simulink model "c960x4096_x14_7_r2013b_frb"  (R2013b)
settings: Solver=ode45  StartTime=0.0  StopTime=40960  RelTol=1e-3
undefined symbols (not defined in the file): sfp
libraries: xbsIndex_r4 x14620, casper_library_misc x61, dspsigops x32, casper_library_multipliers x24, simulink x18, xps_library x18
(part 17 of 79)

== system c960x4096_x14_7_r2013b_frb/ds_to_tgbe/mb1/mb_5 ==
  DIN_0 : Inport
  DIN_1 : Inport  Port=2
  DIN_2 : Inport  Port=3
  DIN_3 : Inport  Port=4
  W_ADDR : Inport  Port=5
  R_ADDR : Inport  Port=6
  WE : Inport  Port=7
  MUX_SEL : Inport  Port=8
  Concat{,1..3} (4 alike) : xbsIndex_r4/Concat  num_inputs=2  dbl_ovrd=off  block_type=concat
  Mux1 : xbsIndex_r4/Mux  inputs=4  en=off  latency=0  precision=Full  arith_type=Unsigned  n_bits=16  bin_pt=14  quantization=Truncate  overflow=Wrap  dbl_ovrd=off  block_type=mux
  Mux2 : xbsIndex_r4/Mux  inputs=2  en=off  latency=0  precision=Full  arith_type=Unsigned  n_bits=16  bin_pt=14  quantization=Truncate  overflow=Wrap  dbl_ovrd=off  block_type=mux
  Slice_Data_0 : Subsystem
  Slice_Data_1 : Subsystem
  Slice_Data_2 : Subsystem
  Slice_Data_3 : Subsystem
  b0h : Subsystem  Tag=xps:bram  AncestorBlock=xps_library/Shared BRAM  mask{arith_type=Unsigned, addr_width=10, data_width=32, reg_prim_output=off, reg_core_output=off, optimization=Minimum_Area, data_bin_pt=0, init_vals=[0:0], sample_rate=1}
      mask prompts: arith_type "Output Data Type"; addr_width "Address width"; data_width "Data Width"; reg_prim_output "Register Primitive Output"; reg_core_output "Register Core Output"; data_bin_pt "Data Binary Point"; init_vals "Initial values (simulation only)"; sample_rate "Sample rate"
      mask init:
      | shared_bram_mask;
      mask TypeOptions arith_type: Unsigned | Signed  (2's comp)
      mask TypeOptions data_width: 8 | 16 | 32 | 64 | 128
      mask TypeOptions optimization: Minimum_Area | Low_Power
  b0l : Subsystem  Tag=xps:bram  AncestorBlock=xps_library/Shared BRAM  mask{arith_type=Unsigned, addr_width=10, data_width=32, reg_prim_output=off, reg_core_output=off, optimization=Minimum_Area, data_bin_pt=0, init_vals=[0:0], sample_rate=1}
      mask prompts: arith_type "Output Data Type"; addr_width "Address width"; data_width "Data Width"; reg_prim_output "Register Primitive Output"; reg_core_output "Register Core Output"; data_bin_pt "Data Binary Point"; init_vals "Initial values (simulation only)"; sample_rate "Sample rate"
      mask init:
      | shared_bram_mask;
      mask TypeOptions arith_type: Unsigned | Signed  (2's comp)
      mask TypeOptions data_width: 8 | 16 | 32 | 64 | 128
      mask TypeOptions optimization: Minimum_Area | Low_Power
  b1h : Subsystem  Tag=xps:bram  AncestorBlock=xps_library/Shared BRAM  mask{arith_type=Unsigned, addr_width=10, data_width=32, reg_prim_output=off, reg_core_output=off, optimization=Minimum_Area, data_bin_pt=0, init_vals=[0:0], sample_rate=1}
      mask prompts: arith_type "Output Data Type"; addr_width "Address width"; data_width "Data Width"; reg_prim_output "Register Primitive Output"; reg_core_output "Register Core Output"; data_bin_pt "Data Binary Point"; init_vals "Initial values (simulation only)"; sample_rate "Sample rate"
      mask init:
      | shared_bram_mask;
      mask TypeOptions arith_type: Unsigned | Signed  (2's comp)
      mask TypeOptions data_width: 8 | 16 | 32 | 64 | 128
      mask TypeOptions optimization: Minimum_Area | Low_Power
  b1l : Subsystem  Tag=xps:bram  AncestorBlock=xps_library/Shared BRAM  mask{arith_type=Unsigned, addr_width=10, data_width=32, reg_prim_output=off, reg_core_output=off, optimization=Minimum_Area, data_bin_pt=0, init_vals=[0:0], sample_rate=1}
      mask prompts: arith_type "Output Data Type"; addr_width "Address width"; data_width "Data Width"; reg_prim_output "Register Primitive Output"; reg_core_output "Register Core Output"; data_bin_pt "Data Binary Point"; init_vals "Initial values (simulation only)"; sample_rate "Sample rate"
      mask init:
      | shared_bram_mask;
      mask TypeOptions arith_type: Unsigned | Signed  (2's comp)
      mask TypeOptions data_width: 8 | 16 | 32 | 64 | 128
      mask TypeOptions optimization: Minimum_Area | Low_Power
  b2h : Subsystem  Tag=xps:bram  AncestorBlock=xps_library/Shared BRAM  mask{arith_type=Unsigned, addr_width=10, data_width=32, reg_prim_output=off, reg_core_output=off, optimization=Minimum_Area, data_bin_pt=0, init_vals=[0:0], sample_rate=1}
      mask prompts: arith_type "Output Data Type"; addr_width "Address width"; data_width "Data Width"; reg_prim_output "Register Primitive Output"; reg_core_output "Register Core Output"; data_bin_pt "Data Binary Point"; init_vals "Initial values (simulation only)"; sample_rate "Sample rate"
      mask init:
      | shared_bram_mask;
      mask TypeOptions arith_type: Unsigned | Signed  (2's comp)
      mask TypeOptions data_width: 8 | 16 | 32 | 64 | 128
      mask TypeOptions optimization: Minimum_Area | Low_Power
  b2l : Subsystem  Tag=xps:bram  AncestorBlock=xps_library/Shared BRAM  mask{arith_type=Unsigned, addr_width=10, data_width=32, reg_prim_output=off, reg_core_output=off, optimization=Minimum_Area, data_bin_pt=0, init_vals=[0:0], sample_rate=1}
      mask prompts: arith_type "Output Data Type"; addr_width "Address width"; data_width "Data Width"; reg_prim_output "Register Primitive Output"; reg_core_output "Register Core Output"; data_bin_pt "Data Binary Point"; init_vals "Initial values (simulation only)"; sample_rate "Sample rate"
      mask init:
      | shared_bram_mask;
      mask TypeOptions arith_type: Unsigned | Signed  (2's comp)
      mask TypeOptions data_width: 8 | 16 | 32 | 64 | 128
      mask TypeOptions optimization: Minimum_Area | Low_Power
  b3h : Subsystem  Tag=xps:bram  AncestorBlock=xps_library/Shared BRAM  mask{arith_type=Unsigned, addr_width=10, data_width=32, reg_prim_output=off, reg_core_output=off, optimization=Minimum_Area, data_bin_pt=0, init_vals=[0:0], sample_rate=1}
      mask prompts: arith_type "Output Data Type"; addr_width "Address width"; data_width "Data Width"; reg_prim_output "Register Primitive Output"; reg_core_output "Register Core Output"; data_bin_pt "Data Binary Point"; init_vals "Initial values (simulation only)"; sample_rate "Sample rate"
      mask init:
      | shared_bram_mask;
      mask TypeOptions arith_type: Unsigned | Signed  (2's comp)
      mask TypeOptions data_width: 8 | 16 | 32 | 64 | 128
      mask TypeOptions optimization: Minimum_Area | Low_Power
  b3l : Subsystem  Tag=xps:bram  AncestorBlock=xps_library/Shared BRAM  mask{arith_type=Unsigned, addr_width=10, data_width=32, reg_prim_output=off, reg_core_output=off, optimization=Minimum_Area, data_bin_pt=0, init_vals=[0:0], sample_rate=1}
      mask prompts: arith_type "Output Data Type"; addr_width "Address width"; data_width "Data Width"; reg_prim_output "Register Primitive Output"; reg_core_output "Register Core Output"; data_bin_pt "Data Binary Point"; init_vals "Initial values (simulation only)"; sample_rate "Sample rate"
      mask init:
      | shared_bram_mask;
      mask TypeOptions arith_type: Unsigned | Signed  (2's comp)
      mask TypeOptions data_width: 8 | 16 | 32 | 64 | 128
      mask TypeOptions optimization: Minimum_Area | Low_Power
  DOUT : Outport
  wires:
  b0h/1(data_out) -> Concat/1
  [R_ADDR] -> Mux2/2
  [W_ADDR] -> Mux2/3
  [WE] -> Mux2/1
  Mux2/1 -> [ADDR]
  R_ADDR/1 -> [R_ADDR]
  Mux1/1 -> DOUT/1
  Concat3/1 -> [MB_3]
  Concat2/1 -> [MB_2]
  Concat1/1 -> [MB_1]
  Concat/1 -> [MB_0]
  [MB_3] -> Mux1/5
  [MB_2] -> Mux1/4
  [MB_1] -> Mux1/3
  [MB_0] -> Mux1/2
  [MUX_SEL] -> Mux1/1
  [ADDR] -> b3l/1(addr), b3h/1(addr), b2l/1(addr), b2h/1(addr), b1l/1(addr), b1h/1(addr), b0l/1(addr), b0h/1(addr)
  [DIN_3] -> Slice_Data_3/1(DIN)
  [DIN_2] -> Slice_Data_2/1(DIN)
  [DIN_1] -> Slice_Data_1/1(DIN)
  [DIN_0] -> Slice_Data_0/1(DIN)
  Slice_Data_3/2(DOUT_LO) -> b3l/2(data_in)
  Slice_Data_3/1(DOUT_HI) -> b3h/2(data_in)
  Slice_Data_2/2(DOUT_LO) -> b2l/2(data_in)
  Slice_Data_2/1(DOUT_HI) -> b2h/2(data_in)
  Slice_Data_1/2(DOUT_LO) -> b1l/2(data_in)
  Slice_Data_1/1(DOUT_HI) -> b1h/2(data_in)
  Slice_Data_0/2(DOUT_LO) -> b0l/2(data_in)
  Slice_Data_0/1(DOUT_HI) -> b0h/2(data_in)
  [WE] -> b3l/3(we), b3h/3(we), b2l/3(we), b2h/3(we), b1l/3(we), b1h/3(we), b0l/3(we), b0h/3(we)
  b3l/1(data_out) -> Concat3/2
  b3h/1(data_out) -> Concat3/1
  b2l/1(data_out) -> Concat2/2
  b2h/1(data_out) -> Concat2/1
  b1l/1(data_out) -> Concat1/2
  b1h/1(data_out) -> Concat1/1
  b0l/1(data_out) -> Concat/2
  MUX_SEL/1 -> [MUX_SEL]
  WE/1 -> [WE]
  W_ADDR/1 -> [W_ADDR]
  DIN_3/1 -> [DIN_3]
  DIN_2/1 -> [DIN_2]
  DIN_1/1 -> [DIN_1]
  DIN_0/1 -> [DIN_0]

== system c960x4096_x14_7_r2013b_frb/ds_to_tgbe/mb1/mb_6 ==
  DIN_0 : Inport
  DIN_1 : Inport  Port=2
  DIN_2 : Inport  Port=3
  DIN_3 : Inport  Port=4
  W_ADDR : Inport  Port=5
  R_ADDR : Inport  Port=6
  WE : Inport  Port=7
  MUX_SEL : Inport  Port=8
  Concat{,1..3} (4 alike) : xbsIndex_r4/Concat  num_inputs=2  dbl_ovrd=off  block_type=concat
  Mux1 : xbsIndex_r4/Mux  inputs=4  en=off  latency=0  precision=Full  arith_type=Unsigned  n_bits=16  bin_pt=14  quantization=Truncate  overflow=Wrap  dbl_ovrd=off  block_type=mux
  Mux2 : xbsIndex_r4/Mux  inputs=2  en=off  latency=0  precision=Full  arith_type=Unsigned  n_bits=16  bin_pt=14  quantization=Truncate  overflow=Wrap  dbl_ovrd=off  block_type=mux
  Slice_Data_0 : Subsystem
  Slice_Data_1 : Subsystem
  Slice_Data_2 : Subsystem
  Slice_Data_3 : Subsystem
  b0h : Subsystem  Tag=xps:bram  AncestorBlock=xps_library/Shared BRAM  mask{arith_type=Unsigned, addr_width=10, data_width=32, reg_prim_output=off, reg_core_output=off, optimization=Minimum_Area, data_bin_pt=0, init_vals=[0:0], sample_rate=1}
      mask prompts: arith_type "Output Data Type"; addr_width "Address width"; data_width "Data Width"; reg_prim_output "Register Primitive Output"; reg_core_output "Register Core Output"; data_bin_pt "Data Binary Point"; init_vals "Initial values (simulation only)"; sample_rate "Sample rate"
      mask init:
      | shared_bram_mask;
      mask TypeOptions arith_type: Unsigned | Signed  (2's comp)
      mask TypeOptions data_width: 8 | 16 | 32 | 64 | 128
      mask TypeOptions optimization: Minimum_Area | Low_Power
  b0l : Subsystem  Tag=xps:bram  AncestorBlock=xps_library/Shared BRAM  mask{arith_type=Unsigned, addr_width=10, data_width=32, reg_prim_output=off, reg_core_output=off, optimization=Minimum_Area, data_bin_pt=0, init_vals=[0:0], sample_rate=1}
      mask prompts: arith_type "Output Data Type"; addr_width "Address width"; data_width "Data Width"; reg_prim_output "Register Primitive Output"; reg_core_output "Register Core Output"; data_bin_pt "Data Binary Point"; init_vals "Initial values (simulation only)"; sample_rate "Sample rate"
      mask init:
      | shared_bram_mask;
      mask TypeOptions arith_type: Unsigned | Signed  (2's comp)
      mask TypeOptions data_width: 8 | 16 | 32 | 64 | 128
      mask TypeOptions optimization: Minimum_Area | Low_Power
  b1h : Subsystem  Tag=xps:bram  AncestorBlock=xps_library/Shared BRAM  mask{arith_type=Unsigned, addr_width=10, data_width=32, reg_prim_output=off, reg_core_output=off, optimization=Minimum_Area, data_bin_pt=0, init_vals=[0:0], sample_rate=1}
      mask prompts: arith_type "Output Data Type"; addr_width "Address width"; data_width "Data Width"; reg_prim_output "Register Primitive Output"; reg_core_output "Register Core Output"; data_bin_pt "Data Binary Point"; init_vals "Initial values (simulation only)"; sample_rate "Sample rate"
      mask init:
      | shared_bram_mask;
      mask TypeOptions arith_type: Unsigned | Signed  (2's comp)
      mask TypeOptions data_width: 8 | 16 | 32 | 64 | 128
      mask TypeOptions optimization: Minimum_Area | Low_Power
  b1l : Subsystem  Tag=xps:bram  AncestorBlock=xps_library/Shared BRAM  mask{arith_type=Unsigned, addr_width=10, data_width=32, reg_prim_output=off, reg_core_output=off, optimization=Minimum_Area, data_bin_pt=0, init_vals=[0:0], sample_rate=1}
      mask prompts: arith_type "Output Data Type"; addr_width "Address width"; data_width "Data Width"; reg_prim_output "Register Primitive Output"; reg_core_output "Register Core Output"; data_bin_pt "Data Binary Point"; init_vals "Initial values (simulation only)"; sample_rate "Sample rate"
      mask init:
      | shared_bram_mask;
      mask TypeOptions arith_type: Unsigned | Signed  (2's comp)
      mask TypeOptions data_width: 8 | 16 | 32 | 64 | 128
      mask TypeOptions optimization: Minimum_Area | Low_Power
  b2h : Subsystem  Tag=xps:bram  AncestorBlock=xps_library/Shared BRAM  mask{arith_type=Unsigned, addr_width=10, data_width=32, reg_prim_output=off, reg_core_output=off, optimization=Minimum_Area, data_bin_pt=0, init_vals=[0:0], sample_rate=1}
      mask prompts: arith_type "Output Data Type"; addr_width "Address width"; data_width "Data Width"; reg_prim_output "Register Primitive Output"; reg_core_output "Register Core Output"; data_bin_pt "Data Binary Point"; init_vals "Initial values (simulation only)"; sample_rate "Sample rate"
      mask init:
      | shared_bram_mask;
      mask TypeOptions arith_type: Unsigned | Signed  (2's comp)
      mask TypeOptions data_width: 8 | 16 | 32 | 64 | 128
      mask TypeOptions optimization: Minimum_Area | Low_Power
  b2l : Subsystem  Tag=xps:bram  AncestorBlock=xps_library/Shared BRAM  mask{arith_type=Unsigned, addr_width=10, data_width=32, reg_prim_output=off, reg_core_output=off, optimization=Minimum_Area, data_bin_pt=0, init_vals=[0:0], sample_rate=1}
      mask prompts: arith_type "Output Data Type"; addr_width "Address width"; data_width "Data Width"; reg_prim_output "Register Primitive Output"; reg_core_output "Register Core Output"; data_bin_pt "Data Binary Point"; init_vals "Initial values (simulation only)"; sample_rate "Sample rate"
      mask init:
      | shared_bram_mask;
      mask TypeOptions arith_type: Unsigned | Signed  (2's comp)
      mask TypeOptions data_width: 8 | 16 | 32 | 64 | 128
      mask TypeOptions optimization: Minimum_Area | Low_Power
  b3h : Subsystem  Tag=xps:bram  AncestorBlock=xps_library/Shared BRAM  mask{arith_type=Unsigned, addr_width=10, data_width=32, reg_prim_output=off, reg_core_output=off, optimization=Minimum_Area, data_bin_pt=0, init_vals=[0:0], sample_rate=1}
      mask prompts: arith_type "Output Data Type"; addr_width "Address width"; data_width "Data Width"; reg_prim_output "Register Primitive Output"; reg_core_output "Register Core Output"; data_bin_pt "Data Binary Point"; init_vals "Initial values (simulation only)"; sample_rate "Sample rate"
      mask init:
      | shared_bram_mask;
      mask TypeOptions arith_type: Unsigned | Signed  (2's comp)
      mask TypeOptions data_width: 8 | 16 | 32 | 64 | 128
      mask TypeOptions optimization: Minimum_Area | Low_Power
  b3l : Subsystem  Tag=xps:bram  AncestorBlock=xps_library/Shared BRAM  mask{arith_type=Unsigned, addr_width=10, data_width=32, reg_prim_output=off, reg_core_output=off, optimization=Minimum_Area, data_bin_pt=0, init_vals=[0:0], sample_rate=1}
      mask prompts: arith_type "Output Data Type"; addr_width "Address width"; data_width "Data Width"; reg_prim_output "Register Primitive Output"; reg_core_output "Register Core Output"; data_bin_pt "Data Binary Point"; init_vals "Initial values (simulation only)"; sample_rate "Sample rate"
      mask init:
      | shared_bram_mask;
      mask TypeOptions arith_type: Unsigned | Signed  (2's comp)
      mask TypeOptions data_width: 8 | 16 | 32 | 64 | 128
      mask TypeOptions optimization: Minimum_Area | Low_Power
  DOUT : Outport
  wires:
  b0h/1(data_out) -> Concat/1
  [R_ADDR] -> Mux2/2
  [W_ADDR] -> Mux2/3
  [WE] -> Mux2/1
  Mux2/1 -> [ADDR]
  R_ADDR/1 -> [R_ADDR]
  Mux1/1 -> DOUT/1
  Concat3/1 -> [MB_3]
  Concat2/1 -> [MB_2]
  Concat1/1 -> [MB_1]
  Concat/1 -> [MB_0]
  [MB_3] -> Mux1/5
  [MB_2] -> Mux1/4
  [MB_1] -> Mux1/3
  [MB_0] -> Mux1/2
  [MUX_SEL] -> Mux1/1
  [ADDR] -> b3l/1(addr), b3h/1(addr), b2l/1(addr), b2h/1(addr), b1l/1(addr), b1h/1(addr), b0l/1(addr), b0h/1(addr)
  [DIN_3] -> Slice_Data_3/1(DIN)
  [DIN_2] -> Slice_Data_2/1(DIN)
  [DIN_1] -> Slice_Data_1/1(DIN)
  [DIN_0] -> Slice_Data_0/1(DIN)
  Slice_Data_3/2(DOUT_LO) -> b3l/2(data_in)
  Slice_Data_3/1(DOUT_HI) -> b3h/2(data_in)
  Slice_Data_2/2(DOUT_LO) -> b2l/2(data_in)
  Slice_Data_2/1(DOUT_HI) -> b2h/2(data_in)
  Slice_Data_1/2(DOUT_LO) -> b1l/2(data_in)
  Slice_Data_1/1(DOUT_HI) -> b1h/2(data_in)
  Slice_Data_0/2(DOUT_LO) -> b0l/2(data_in)
  Slice_Data_0/1(DOUT_HI) -> b0h/2(data_in)
  [WE] -> b3l/3(we), b3h/3(we), b2l/3(we), b2h/3(we), b1l/3(we), b1h/3(we), b0l/3(we), b0h/3(we)
  b3l/1(data_out) -> Concat3/2
  b3h/1(data_out) -> Concat3/1
  b2l/1(data_out) -> Concat2/2
  b2h/1(data_out) -> Concat2/1
  b1l/1(data_out) -> Concat1/2
  b1h/1(data_out) -> Concat1/1
  b0l/1(data_out) -> Concat/2
  MUX_SEL/1 -> [MUX_SEL]
  WE/1 -> [WE]
  W_ADDR/1 -> [W_ADDR]
  DIN_3/1 -> [DIN_3]
  DIN_2/1 -> [DIN_2]
  DIN_1/1 -> [DIN_1]
  DIN_0/1 -> [DIN_0]

== system c960x4096_x14_7_r2013b_frb/ds_to_tgbe/mb1/mb_7 ==
  DIN_0 : Inport
  DIN_1 : Inport  Port=2
  DIN_2 : Inport  Port=3
  DIN_3 : Inport  Port=4
  W_ADDR : Inport  Port=5
  R_ADDR : Inport  Port=6
  WE : Inport  Port=7
  MUX_SEL : Inport  Port=8
  Concat{,1..3} (4 alike) : xbsIndex_r4/Concat  num_inputs=2  dbl_ovrd=off  block_type=concat
  Mux1 : xbsIndex_r4/Mux  inputs=4  en=off  latency=0  precision=Full  arith_type=Unsigned  n_bits=16  bin_pt=14  quantization=Truncate  overflow=Wrap  dbl_ovrd=off  block_type=mux
  Mux2 : xbsIndex_r4/Mux  inputs=2  en=off  latency=0  precision=Full  arith_type=Unsigned  n_bits=16  bin_pt=14  quantization=Truncate  overflow=Wrap  dbl_ovrd=off  block_type=mux
  Slice_Data_0 : Subsystem
  Slice_Data_1 : Subsystem
  Slice_Data_2 : Subsystem
  Slice_Data_3 : Subsystem
  b0h : Subsystem  Tag=xps:bram  AncestorBlock=xps_library/Shared BRAM  mask{arith_type=Unsigned, addr_width=10, data_width=32, reg_prim_output=off, reg_core_output=off, optimization=Minimum_Area, data_bin_pt=0, init_vals=[0:0], sample_rate=1}
      mask prompts: arith_type "Output Data Type"; addr_width "Address width"; data_width "Data Width"; reg_prim_output "Register Primitive Output"; reg_core_output "Register Core Output"; data_bin_pt "Data Binary Point"; init_vals "Initial values (simulation only)"; sample_rate "Sample rate"
      mask init:
      | shared_bram_mask;
      mask TypeOptions arith_type: Unsigned | Signed  (2's comp)
      mask TypeOptions data_width: 8 | 16 | 32 | 64 | 128
      mask TypeOptions optimization: Minimum_Area | Low_Power
  b0l : Subsystem  Tag=xps:bram  AncestorBlock=xps_library/Shared BRAM  mask{arith_type=Unsigned, addr_width=10, data_width=32, reg_prim_output=off, reg_core_output=off, optimization=Minimum_Area, data_bin_pt=0, init_vals=[0:0], sample_rate=1}
      mask prompts: arith_type "Output Data Type"; addr_width "Address width"; data_width "Data Width"; reg_prim_output "Register Primitive Output"; reg_core_output "Register Core Output"; data_bin_pt "Data Binary Point"; init_vals "Initial values (simulation only)"; sample_rate "Sample rate"
      mask init:
      | shared_bram_mask;
      mask TypeOptions arith_type: Unsigned | Signed  (2's comp)
      mask TypeOptions data_width: 8 | 16 | 32 | 64 | 128
      mask TypeOptions optimization: Minimum_Area | Low_Power
  b1h : Subsystem  Tag=xps:bram  AncestorBlock=xps_library/Shared BRAM  mask{arith_type=Unsigned, addr_width=10, data_width=32, reg_prim_output=off, reg_core_output=off, optimization=Minimum_Area, data_bin_pt=0, init_vals=[0:0], sample_rate=1}
      mask prompts: arith_type "Output Data Type"; addr_width "Address width"; data_width "Data Width"; reg_prim_output "Register Primitive Output"; reg_core_output "Register Core Output"; data_bin_pt "Data Binary Point"; init_vals "Initial values (simulation only)"; sample_rate "Sample rate"
      mask init:
      | shared_bram_mask;
      mask TypeOptions arith_type: Unsigned | Signed  (2's comp)
      mask TypeOptions data_width: 8 | 16 | 32 | 64 | 128
      mask TypeOptions optimization: Minimum_Area | Low_Power
  b1l : Subsystem  Tag=xps:bram  AncestorBlock=xps_library/Shared BRAM  mask{arith_type=Unsigned, addr_width=10, data_width=32, reg_prim_output=off, reg_core_output=off, optimization=Minimum_Area, data_bin_pt=0, init_vals=[0:0], sample_rate=1}
      mask prompts: arith_type "Output Data Type"; addr_width "Address width"; data_width "Data Width"; reg_prim_output "Register Primitive Output"; reg_core_output "Register Core Output"; data_bin_pt "Data Binary Point"; init_vals "Initial values (simulation only)"; sample_rate "Sample rate"
      mask init:
      | shared_bram_mask;
      mask TypeOptions arith_type: Unsigned | Signed  (2's comp)
      mask TypeOptions data_width: 8 | 16 | 32 | 64 | 128
      mask TypeOptions optimization: Minimum_Area | Low_Power
  b2h : Subsystem  Tag=xps:bram  AncestorBlock=xps_library/Shared BRAM  mask{arith_type=Unsigned, addr_width=10, data_width=32, reg_prim_output=off, reg_core_output=off, optimization=Minimum_Area, data_bin_pt=0, init_vals=[0:0], sample_rate=1}
      mask prompts: arith_type "Output Data Type"; addr_width "Address width"; data_width "Data Width"; reg_prim_output "Register Primitive Output"; reg_core_output "Register Core Output"; data_bin_pt "Data Binary Point"; init_vals "Initial values (simulation only)"; sample_rate "Sample rate"
      mask init:
      | shared_bram_mask;
      mask TypeOptions arith_type: Unsigned | Signed  (2's comp)
      mask TypeOptions data_width: 8 | 16 | 32 | 64 | 128
      mask TypeOptions optimization: Minimum_Area | Low_Power
  b2l : Subsystem  Tag=xps:bram  AncestorBlock=xps_library/Shared BRAM  mask{arith_type=Unsigned, addr_width=10, data_width=32, reg_prim_output=off, reg_core_output=off, optimization=Minimum_Area, data_bin_pt=0, init_vals=[0:0], sample_rate=1}
      mask prompts: arith_type "Output Data Type"; addr_width "Address width"; data_width "Data Width"; reg_prim_output "Register Primitive Output"; reg_core_output "Register Core Output"; data_bin_pt "Data Binary Point"; init_vals "Initial values (simulation only)"; sample_rate "Sample rate"
      mask init:
      | shared_bram_mask;
      mask TypeOptions arith_type: Unsigned | Signed  (2's comp)
      mask TypeOptions data_width: 8 | 16 | 32 | 64 | 128
      mask TypeOptions optimization: Minimum_Area | Low_Power
  b3h : Subsystem  Tag=xps:bram  AncestorBlock=xps_library/Shared BRAM  mask{arith_type=Unsigned, addr_width=10, data_width=32, reg_prim_output=off, reg_core_output=off, optimization=Minimum_Area, data_bin_pt=0, init_vals=[0:0], sample_rate=1}
      mask prompts: arith_type "Output Data Type"; addr_width "Address width"; data_width "Data Width"; reg_prim_output "Register Primitive Output"; reg_core_output "Register Core Output"; data_bin_pt "Data Binary Point"; init_vals "Initial values (simulation only)"; sample_rate "Sample rate"
      mask init:
      | shared_bram_mask;
      mask TypeOptions arith_type: Unsigned | Signed  (2's comp)
      mask TypeOptions data_width: 8 | 16 | 32 | 64 | 128
      mask TypeOptions optimization: Minimum_Area | Low_Power
  b3l : Subsystem  Tag=xps:bram  AncestorBlock=xps_library/Shared BRAM  mask{arith_type=Unsigned, addr_width=10, data_width=32, reg_prim_output=off, reg_core_output=off, optimization=Minimum_Area, data_bin_pt=0, init_vals=[0:0], sample_rate=1}
      mask prompts: arith_type "Output Data Type"; addr_width "Address width"; data_width "Data Width"; reg_prim_output "Register Primitive Output"; reg_core_output "Register Core Output"; data_bin_pt "Data Binary Point"; init_vals "Initial values (simulation only)"; sample_rate "Sample rate"
      mask init:
      | shared_bram_mask;
      mask TypeOptions arith_type: Unsigned | Signed  (2's comp)
      mask TypeOptions data_width: 8 | 16 | 32 | 64 | 128
      mask TypeOptions optimization: Minimum_Area | Low_Power
  DOUT : Outport
  wires:
  b0h/1(data_out) -> Concat/1
  [R_ADDR] -> Mux2/2
  [W_ADDR] -> Mux2/3
  [WE] -> Mux2/1
  Mux2/1 -> [ADDR]
  R_ADDR/1 -> [R_ADDR]
  Mux1/1 -> DOUT/1
  Concat3/1 -> [MB_3]
  Concat2/1 -> [MB_2]
  Concat1/1 -> [MB_1]
  Concat/1 -> [MB_0]
  [MB_3] -> Mux1/5
  [MB_2] -> Mux1/4
  [MB_1] -> Mux1/3
  [MB_0] -> Mux1/2
  [MUX_SEL] -> Mux1/1
  [ADDR] -> b3l/1(addr), b3h/1(addr), b2l/1(addr), b2h/1(addr), b1l/1(addr), b1h/1(addr), b0l/1(addr), b0h/1(addr)
  [DIN_3] -> Slice_Data_3/1(DIN)
  [DIN_2] -> Slice_Data_2/1(DIN)
  [DIN_1] -> Slice_Data_1/1(DIN)
  [DIN_0] -> Slice_Data_0/1(DIN)
  Slice_Data_3/2(DOUT_LO) -> b3l/2(data_in)
  Slice_Data_3/1(DOUT_HI) -> b3h/2(data_in)
  Slice_Data_2/2(DOUT_LO) -> b2l/2(data_in)
  Slice_Data_2/1(DOUT_HI) -> b2h/2(data_in)
  Slice_Data_1/2(DOUT_LO) -> b1l/2(data_in)
  Slice_Data_1/1(DOUT_HI) -> b1h/2(data_in)
  Slice_Data_0/2(DOUT_LO) -> b0l/2(data_in)
  Slice_Data_0/1(DOUT_HI) -> b0h/2(data_in)
  [WE] -> b3l/3(we), b3h/3(we), b2l/3(we), b2h/3(we), b1l/3(we), b1h/3(we), b0l/3(we), b0h/3(we)
  b3l/1(data_out) -> Concat3/2
  b3h/1(data_out) -> Concat3/1
  b2l/1(data_out) -> Concat2/2
  b2h/1(data_out) -> Concat2/1
  b1l/1(data_out) -> Concat1/2
  b1h/1(data_out) -> Concat1/1
  b0l/1(data_out) -> Concat/2
  MUX_SEL/1 -> [MUX_SEL]
  WE/1 -> [WE]
  W_ADDR/1 -> [W_ADDR]
  DIN_3/1 -> [DIN_3]
  DIN_2/1 -> [DIN_2]
  DIN_1/1 -> [DIN_1]
  DIN_0/1 -> [DIN_0]

== system c960x4096_x14_7_r2013b_frb/ds_to_tgbe/mb_rd/MSYNC_TREE ==
  In1 : Inport
  Register{1,3,5..6,9,11,41..43,45..46} (11 alike) : xbsIndex_r4/Register  init=0  rst=off  en=off  dbl_ovrd=off  block_type=register
      settings: block_version=11.4
  Out1 : Outport
  Out2 : Outport  Port=2
  Out3 : Outport  Port=3
  Out4 : Outport  Port=4
  Out5 : Outport  Port=5
  Out6 : Outport  Port=6
  Out7 : Outport  Port=7
  Out8 : Outport  Port=8
  wires:
  In1/1 -> Register41/1
  Register43/1 -> Out1/1
  Register41/1 -> Register45/1, Register42/1
  Register11/1 -> Out8/1
  Register9/1 -> Out7/1
  Register5/1 -> Out6/1
  Register3/1 -> Out5/1
  Register1/1 -> Out4/1
  Register6/1 -> Out3/1
  Register46/1 -> Out2/1
  Register42/1 -> Register46/1, Register6/1, Register1/1, Register43/1
  Register45/1 -> Register5/1, Register9/1, Register11/1, Register3/1

== system c960x4096_x14_7_r2013b_frb/ds_to_tgbe/mb_rd/NCHAN_TREE ==
  In1 : Inport
  Register{1,3,5..6,9,11,41..43,45..46} (11 alike) : xbsIndex_r4/Register  init=0  rst=off  en=off  dbl_ovrd=off  block_type=register
      settings: block_version=11.4
  Out1 : Outport
  Out2 : Outport  Port=2
  Out3 : Outport  Port=3
  Out4 : Outport  Port=4
  Out5 : Outport  Port=5
  Out6 : Outport  Port=6
  Out7 : Outport  Port=7
  Out8 : Outport  Port=8
  wires:
  In1/1 -> Register41/1
  Register43/1 -> Out1/1
  Register41/1 -> Register45/1, Register42/1
  Register11/1 -> Out8/1
  Register9/1 -> Out7/1
  Register5/1 -> Out6/1
  Register3/1 -> Out5/1
  Register1/1 -> Out4/1
  Register6/1 -> Out3/1
  Register46/1 -> Out2/1
  Register42/1 -> Register46/1, Register6/1, Register1/1, Register43/1
  Register45/1 -> Register5/1, Register9/1, Register11/1, Register3/1

== system c960x4096_x14_7_r2013b_frb/ds_to_tgbe/mb_rd/XFER_0 ==
  MSYNC : Inport
  NCHAN : Inport  Port=2
  DIN : Inport  Port=3
  WE : Inport  Port=4
  NODE_ID : Inport  Port=5
  FEC : Inport  Port=6
  IFG0 : Inport  Port=7
  IFG1 : Inport  Port=8
  GEN_ENC_FC : Subsystem
  GEN_R_ADDR_MUX_SEL : Subsystem
  GEN_STB_EOF_W_COUNT : Subsystem
  OUTPUT_MUX : Subsystem
  R_ADDR : Outport
  MUX_SEL : Outport  Port=2
  DOUT : Outport  Port=3
  STB : Outport  Port=4
  EOF : Outport  Port=5
  wires:
  IFG1/1 -> [IFG1]
  IFG0/1 -> [IFG0]
  FEC/1 -> [FEC]
  [EOF] -> EOF/1
  [STB] -> STB/1
  [DOUT] -> DOUT/1
  [MUX_SEL] -> MUX_SEL/1
  [R_ADDR] -> R_ADDR/1
  NODE_ID/1 -> [NODE_ID]
  WE/1 -> [WE]
  DIN/1 -> [DIN]
  NCHAN/1 -> [NCHAN]
  MSYNC/1 -> [MSYNC]
  GEN_R_ADDR_MUX_SEL/2(MUX_SEL) -> [MUX_SEL]
  GEN_R_ADDR_MUX_SEL/1(R_ADDR) -> [R_ADDR]
  OUTPUT_MUX/1(DATA_OUT) -> [DOUT]
  [IFG1] -> OUTPUT_MUX/6(IFG1)
  [IFG0] -> OUTPUT_MUX/5(IFG0)
  [FEC] -> OUTPUT_MUX/4(FEC)
  [NCHAN] -> GEN_R_ADDR_MUX_SEL/3(NCHAN)
  [WE] -> GEN_R_ADDR_MUX_SEL/2(WE)
  [MSYNC] -> GEN_R_ADDR_MUX_SEL/1(MSYNC)
  GEN_STB_EOF_W_COUNT/3(W_COUNT) -> [W_COUNT]
  GEN_STB_EOF_W_COUNT/2(EOF) -> [EOF]
  GEN_STB_EOF_W_COUNT/1(STB) -> [STB]
  [NCHAN] -> GEN_STB_EOF_W_COUNT/3(NCHAN)
  [WE] -> GEN_STB_EOF_W_COUNT/2(WE)
  [MSYNC] -> GEN_STB_EOF_W_COUNT/1(MSYNC)
  [DIN] -> OUTPUT_MUX/3(DATA)
  [ENC_FC] -> OUTPUT_MUX/2(ENC_FC)
  [W_COUNT] -> OUTPUT_MUX/1(W_COUNT)
  GEN_ENC_FC/1(ENC_FC) -> [ENC_FC]
  [EOF] -> GEN_ENC_FC/3(EOF)
  [NODE_ID] -> GEN_ENC_FC/1(NODE_ID)
  [MSYNC] -> GEN_ENC_FC/2(MSYNC)

== system c960x4096_x14_7_r2013b_frb/ds_to_tgbe/mb_rd/XFER_1 ==
  MSYNC : Inport
  NCHAN : Inport  Port=2
  DIN : Inport  Port=3
  WE : Inport  Port=4
  NODE_ID : Inport  Port=5
  FEC : Inport  Port=6
  IFG0 : Inport  Port=7
  IFG1 : Inport  Port=8
  GEN_ENC_FC : Subsystem
  GEN_R_ADDR_MUX_SEL : Subsystem
  GEN_STB_EOF_W_COUNT : Subsystem
  OUTPUT_MUX : Subsystem
  R_ADDR : Outport
  MUX_SEL : Outport  Port=2
  DOUT : Outport  Port=3
  STB : Outport  Port=4
  EOF : Outport  Port=5
  wires:
  IFG1/1 -> [IFG1]
  IFG0/1 -> [IFG0]
  FEC/1 -> [FEC]
  [EOF] -> EOF/1
  [STB] -> STB/1
  [DOUT] -> DOUT/1
  [MUX_SEL] -> MUX_SEL/1
  [R_ADDR] -> R_ADDR/1
  NODE_ID/1 -> [NODE_ID]
  WE/1 -> [WE]
  DIN/1 -> [DIN]
  NCHAN/1 -> [NCHAN]
  MSYNC/1 -> [MSYNC]
  GEN_R_ADDR_MUX_SEL/2(MUX_SEL) -> [MUX_SEL]
  GEN_R_ADDR_MUX_SEL/1(R_ADDR) -> [R_ADDR]
  OUTPUT_MUX/1(DATA_OUT) -> [DOUT]
  [IFG1] -> OUTPUT_MUX/6(IFG1)
  [IFG0] -> OUTPUT_MUX/5(IFG0)
  [FEC] -> OUTPUT_MUX/4(FEC)
  [NCHAN] -> GEN_R_ADDR_MUX_SEL/3(NCHAN)
  [WE] -> GEN_R_ADDR_MUX_SEL/2(WE)
  [MSYNC] -> GEN_R_ADDR_MUX_SEL/1(MSYNC)
  GEN_STB_EOF_W_COUNT/3(W_COUNT) -> [W_COUNT]
  GEN_STB_EOF_W_COUNT/2(EOF) -> [EOF]
  GEN_STB_EOF_W_COUNT/1(STB) -> [STB]
  [NCHAN] -> GEN_STB_EOF_W_COUNT/3(NCHAN)
  [WE] -> GEN_STB_EOF_W_COUNT/2(WE)
  [MSYNC] -> GEN_STB_EOF_W_COUNT/1(MSYNC)
  [DIN] -> OUTPUT_MUX/3(DATA)
  [ENC_FC] -> OUTPUT_MUX/2(ENC_FC)
  [W_COUNT] -> OUTPUT_MUX/1(W_COUNT)
  GEN_ENC_FC/1(ENC_FC) -> [ENC_FC]
  [EOF] -> GEN_ENC_FC/3(EOF)
  [NODE_ID] -> GEN_ENC_FC/1(NODE_ID)
  [MSYNC] -> GEN_ENC_FC/2(MSYNC)

== system c960x4096_x14_7_r2013b_frb/ds_to_tgbe/mb_rd/XFER_2 ==
  MSYNC : Inport
  NCHAN : Inport  Port=2
  DIN : Inport  Port=3
  WE : Inport  Port=4
  NODE_ID : Inport  Port=5
  FEC : Inport  Port=6
  IFG0 : Inport  Port=7
  IFG1 : Inport  Port=8
  GEN_ENC_FC : Subsystem
  GEN_R_ADDR_MUX_SEL : Subsystem
  GEN_STB_EOF_W_COUNT : Subsystem
  OUTPUT_MUX : Subsystem
  R_ADDR : Outport
  MUX_SEL : Outport  Port=2
  DOUT : Outport  Port=3
  STB : Outport  Port=4
  EOF : Outport  Port=5
  wires:
  IFG1/1 -> [IFG1]
  IFG0/1 -> [IFG0]
  FEC/1 -> [FEC]
  [EOF] -> EOF/1
  [STB] -> STB/1
  [DOUT] -> DOUT/1
  [MUX_SEL] -> MUX_SEL/1
  [R_ADDR] -> R_ADDR/1
  NODE_ID/1 -> [NODE_ID]
  WE/1 -> [WE]
  DIN/1 -> [DIN]
  NCHAN/1 -> [NCHAN]
  MSYNC/1 -> [MSYNC]
  GEN_R_ADDR_MUX_SEL/2(MUX_SEL) -> [MUX_SEL]
  GEN_R_ADDR_MUX_SEL/1(R_ADDR) -> [R_ADDR]
  OUTPUT_MUX/1(DATA_OUT) -> [DOUT]
  [IFG1] -> OUTPUT_MUX/6(IFG1)
  [IFG0] -> OUTPUT_MUX/5(IFG0)
  [FEC] -> OUTPUT_MUX/4(FEC)
  [NCHAN] -> GEN_R_ADDR_MUX_SEL/3(NCHAN)
  [WE] -> GEN_R_ADDR_MUX_SEL/2(WE)
  [MSYNC] -> GEN_R_ADDR_MUX_SEL/1(MSYNC)
  GEN_STB_EOF_W_COUNT/3(W_COUNT) -> [W_COUNT]
  GEN_STB_EOF_W_COUNT/2(EOF) -> [EOF]
  GEN_STB_EOF_W_COUNT/1(STB) -> [STB]
  [NCHAN] -> GEN_STB_EOF_W_COUNT/3(NCHAN)
  [WE] -> GEN_STB_EOF_W_COUNT/2(WE)
  [MSYNC] -> GEN_STB_EOF_W_COUNT/1(MSYNC)
  [DIN] -> OUTPUT_MUX/3(DATA)
  [ENC_FC] -> OUTPUT_MUX/2(ENC_FC)
  [W_COUNT] -> OUTPUT_MUX/1(W_COUNT)
  GEN_ENC_FC/1(ENC_FC) -> [ENC_FC]
  [EOF] -> GEN_ENC_FC/3(EOF)
  [NODE_ID] -> GEN_ENC_FC/1(NODE_ID)
  [MSYNC] -> GEN_ENC_FC/2(MSYNC)

== system c960x4096_x14_7_r2013b_frb/ds_to_tgbe/mb_rd/XFER_3 ==
  MSYNC : Inport
  NCHAN : Inport  Port=2
  DIN : Inport  Port=3
  WE : Inport  Port=4
  NODE_ID : Inport  Port=5
  FEC : Inport  Port=6
  IFG0 : Inport  Port=7
  IFG1 : Inport  Port=8
  GEN_ENC_FC : Subsystem
  GEN_R_ADDR_MUX_SEL : Subsystem
  GEN_STB_EOF_W_COUNT : Subsystem
  OUTPUT_MUX : Subsystem
  R_ADDR : Outport
  MUX_SEL : Outport  Port=2
  DOUT : Outport  Port=3
  STB : Outport  Port=4
  EOF : Outport  Port=5
  wires:
  IFG1/1 -> [IFG1]
  IFG0/1 -> [IFG0]
  FEC/1 -> [FEC]
  [EOF] -> EOF/1
  [STB] -> STB/1
  [DOUT] -> DOUT/1
  [MUX_SEL] -> MUX_SEL/1
  [R_ADDR] -> R_ADDR/1
  NODE_ID/1 -> [NODE_ID]
  WE/1 -> [WE]
  DIN/1 -> [DIN]
  NCHAN/1 -> [NCHAN]
  MSYNC/1 -> [MSYNC]
  GEN_R_ADDR_MUX_SEL/2(MUX_SEL) -> [MUX_SEL]
  GEN_R_ADDR_MUX_SEL/1(R_ADDR) -> [R_ADDR]
  OUTPUT_MUX/1(DATA_OUT) -> [DOUT]
  [IFG1] -> OUTPUT_MUX/6(IFG1)
  [IFG0] -> OUTPUT_MUX/5(IFG0)
  [FEC] -> OUTPUT_MUX/4(FEC)
  [NCHAN] -> GEN_R_ADDR_MUX_SEL/3(NCHAN)
  [WE] -> GEN_R_ADDR_MUX_SEL/2(WE)
  [MSYNC] -> GEN_R_ADDR_MUX_SEL/1(MSYNC)
  GEN_STB_EOF_W_COUNT/3(W_COUNT) -> [W_COUNT]
  GEN_STB_EOF_W_COUNT/2(EOF) -> [EOF]
  GEN_STB_EOF_W_COUNT/1(STB) -> [STB]
  [NCHAN] -> GEN_STB_EOF_W_COUNT/3(NCHAN)
  [WE] -> GEN_STB_EOF_W_COUNT/2(WE)
  [MSYNC] -> GEN_STB_EOF_W_COUNT/1(MSYNC)
  [DIN] -> OUTPUT_MUX/3(DATA)
  [ENC_FC] -> OUTPUT_MUX/2(ENC_FC)
  [W_COUNT] -> OUTPUT_MUX/1(W_COUNT)
  GEN_ENC_FC/1(ENC_FC) -> [ENC_FC]
  [EOF] -> GEN_ENC_FC/3(EOF)
  [NODE_ID] -> GEN_ENC_FC/1(NODE_ID)
  [MSYNC] -> GEN_ENC_FC/2(MSYNC)

== system c960x4096_x14_7_r2013b_frb/ds_to_tgbe/mb_rd/XFER_4 ==
  MSYNC : Inport
  NCHAN : Inport  Port=2
  DIN : Inport  Port=3
  WE : Inport  Port=4
  NODE_ID : Inport  Port=5
  FEC : Inport  Port=6
  IFG0 : Inport  Port=7
  IFG1 : Inport  Port=8
  GEN_ENC_FC : Subsystem
  GEN_R_ADDR_MUX_SEL : Subsystem
  GEN_STB_EOF_W_COUNT : Subsystem
  OUTPUT_MUX : Subsystem
  R_ADDR : Outport
  MUX_SEL : Outport  Port=2
  DOUT : Outport  Port=3
  STB : Outport  Port=4
  EOF : Outport  Port=5
  wires:
  IFG1/1 -> [IFG1]
  IFG0/1 -> [IFG0]
  FEC/1 -> [FEC]
  [EOF] -> EOF/1
  [STB] -> STB/1
  [DOUT] -> DOUT/1
  [MUX_SEL] -> MUX_SEL/1
  [R_ADDR] -> R_ADDR/1
  NODE_ID/1 -> [NODE_ID]
  WE/1 -> [WE]
  DIN/1 -> [DIN]
  NCHAN/1 -> [NCHAN]
  MSYNC/1 -> [MSYNC]
  GEN_R_ADDR_MUX_SEL/2(MUX_SEL) -> [MUX_SEL]
  GEN_R_ADDR_MUX_SEL/1(R_ADDR) -> [R_ADDR]
  OUTPUT_MUX/1(DATA_OUT) -> [DOUT]
  [IFG1] -> OUTPUT_MUX/6(IFG1)
  [IFG0] -> OUTPUT_MUX/5(IFG0)
  [FEC] -> OUTPUT_MUX/4(FEC)
  [NCHAN] -> GEN_R_ADDR_MUX_SEL/3(NCHAN)
  [WE] -> GEN_R_ADDR_MUX_SEL/2(WE)
  [MSYNC] -> GEN_R_ADDR_MUX_SEL/1(MSYNC)
  GEN_STB_EOF_W_COUNT/3(W_COUNT) -> [W_COUNT]
  GEN_STB_EOF_W_COUNT/2(EOF) -> [EOF]
  GEN_STB_EOF_W_COUNT/1(STB) -> [STB]
  [NCHAN] -> GEN_STB_EOF_W_COUNT/3(NCHAN)
  [WE] -> GEN_STB_EOF_W_COUNT/2(WE)
  [MSYNC] -> GEN_STB_EOF_W_COUNT/1(MSYNC)
  [DIN] -> OUTPUT_MUX/3(DATA)
  [ENC_FC] -> OUTPUT_MUX/2(ENC_FC)
  [W_COUNT] -> OUTPUT_MUX/1(W_COUNT)
  GEN_ENC_FC/1(ENC_FC) -> [ENC_FC]
  [EOF] -> GEN_ENC_FC/3(EOF)
  [NODE_ID] -> GEN_ENC_FC/1(NODE_ID)
  [MSYNC] -> GEN_ENC_FC/2(MSYNC)

== system c960x4096_x14_7_r2013b_frb/ds_to_tgbe/mb_rd/XFER_5 ==
  MSYNC : Inport
  NCHAN : Inport  Port=2
  DIN : Inport  Port=3
  WE : Inport  Port=4
  NODE_ID : Inport  Port=5
  FEC : Inport  Port=6
  IFG0 : Inport  Port=7
  IFG1 : Inport  Port=8
  GEN_ENC_FC : Subsystem
  GEN_R_ADDR_MUX_SEL : Subsystem
  GEN_STB_EOF_W_COUNT : Subsystem
  OUTPUT_MUX : Subsystem
  R_ADDR : Outport
  MUX_SEL : Outport  Port=2
  DOUT : Outport  Port=3
  STB : Outport  Port=4
  EOF : Outport  Port=5
  wires:
  IFG1/1 -> [IFG1]
  IFG0/1 -> [IFG0]
  FEC/1 -> [FEC]
  [EOF] -> EOF/1
  [STB] -> STB/1
  [DOUT] -> DOUT/1
  [MUX_SEL] -> MUX_SEL/1
  [R_ADDR] -> R_ADDR/1
  NODE_ID/1 -> [NODE_ID]
  WE/1 -> [WE]
  DIN/1 -> [DIN]
  NCHAN/1 -> [NCHAN]
  MSYNC/1 -> [MSYNC]
  GEN_R_ADDR_MUX_SEL/2(MUX_SEL) -> [MUX_SEL]
  GEN_R_ADDR_MUX_SEL/1(R_ADDR) -> [R_ADDR]
  OUTPUT_MUX/1(DATA_OUT) -> [DOUT]
  [IFG1] -> OUTPUT_MUX/6(IFG1)
  [IFG0] -> OUTPUT_MUX/5(IFG0)
  [FEC] -> OUTPUT_MUX/4(FEC)
  [NCHAN] -> GEN_R_ADDR_MUX_SEL/3(NCHAN)
  [WE] -> GEN_R_ADDR_MUX_SEL/2(WE)
  [MSYNC] -> GEN_R_ADDR_MUX_SEL/1(MSYNC)
  GEN_STB_EOF_W_COUNT/3(W_COUNT) -> [W_COUNT]
  GEN_STB_EOF_W_COUNT/2(EOF) -> [EOF]
  GEN_STB_EOF_W_COUNT/1(STB) -> [STB]
  [NCHAN] -> GEN_STB_EOF_W_COUNT/3(NCHAN)
  [WE] -> GEN_STB_EOF_W_COUNT/2(WE)
  [MSYNC] -> GEN_STB_EOF_W_COUNT/1(MSYNC)
  [DIN] -> OUTPUT_MUX/3(DATA)
  [ENC_FC] -> OUTPUT_MUX/2(ENC_FC)
  [W_COUNT] -> OUTPUT_MUX/1(W_COUNT)
  GEN_ENC_FC/1(ENC_FC) -> [ENC_FC]
  [EOF] -> GEN_ENC_FC/3(EOF)
  [NODE_ID] -> GEN_ENC_FC/1(NODE_ID)
  [MSYNC] -> GEN_ENC_FC/2(MSYNC)

== system c960x4096_x14_7_r2013b_frb/ds_to_tgbe/mb_rd/XFER_6 ==
  MSYNC : Inport
  NCHAN : Inport  Port=2
  DIN : Inport  Port=3
  WE : Inport  Port=4
  NODE_ID : Inport  Port=5
  FEC : Inport  Port=6
  IFG0 : Inport  Port=7
  IFG1 : Inport  Port=8
  GEN_ENC_FC : Subsystem
  GEN_R_ADDR_MUX_SEL : Subsystem
  GEN_STB_EOF_W_COUNT : Subsystem
  OUTPUT_MUX : Subsystem
  R_ADDR : Outport
  MUX_SEL : Outport  Port=2
  DOUT : Outport  Port=3
  STB : Outport  Port=4
  EOF : Outport  Port=5
  wires:
  IFG1/1 -> [IFG1]
  IFG0/1 -> [IFG0]
  FEC/1 -> [FEC]
  [EOF] -> EOF/1
  [STB] -> STB/1
  [DOUT] -> DOUT/1
  [MUX_SEL] -> MUX_SEL/1
  [R_ADDR] -> R_ADDR/1
  NODE_ID/1 -> [NODE_ID]
  WE/1 -> [WE]
  DIN/1 -> [DIN]
  NCHAN/1 -> [NCHAN]
  MSYNC/1 -> [MSYNC]
  GEN_R_ADDR_MUX_SEL/2(MUX_SEL) -> [MUX_SEL]
  GEN_R_ADDR_MUX_SEL/1(R_ADDR) -> [R_ADDR]
  OUTPUT_MUX/1(DATA_OUT) -> [DOUT]
  [IFG1] -> OUTPUT_MUX/6(IFG1)
  [IFG0] -> OUTPUT_MUX/5(IFG0)
  [FEC] -> OUTPUT_MUX/4(FEC)
  [NCHAN] -> GEN_R_ADDR_MUX_SEL/3(NCHAN)
  [WE] -> GEN_R_ADDR_MUX_SEL/2(WE)
  [MSYNC] -> GEN_R_ADDR_MUX_SEL/1(MSYNC)
  GEN_STB_EOF_W_COUNT/3(W_COUNT) -> [W_COUNT]
  GEN_STB_EOF_W_COUNT/2(EOF) -> [EOF]
  GEN_STB_EOF_W_COUNT/1(STB) -> [STB]
  [NCHAN] -> GEN_STB_EOF_W_COUNT/3(NCHAN)
  [WE] -> GEN_STB_EOF_W_COUNT/2(WE)
  [MSYNC] -> GEN_STB_EOF_W_COUNT/1(MSYNC)
  [DIN] -> OUTPUT_MUX/3(DATA)
  [ENC_FC] -> OUTPUT_MUX/2(ENC_FC)
  [W_COUNT] -> OUTPUT_MUX/1(W_COUNT)
  GEN_ENC_FC/1(ENC_FC) -> [ENC_FC]
  [EOF] -> GEN_ENC_FC/3(EOF)
  [NODE_ID] -> GEN_ENC_FC/1(NODE_ID)
  [MSYNC] -> GEN_ENC_FC/2(MSYNC)

== system c960x4096_x14_7_r2013b_frb/ds_to_tgbe/mb_rd/XFER_7 ==
  MSYNC : Inport
  NCHAN : Inport  Port=2
  DIN : Inport  Port=3
  WE : Inport  Port=4
  NODE_ID : Inport  Port=5
  FEC : Inport  Port=6
  IFG0 : Inport  Port=7
  IFG1 : Inport  Port=8
  GEN_ENC_FC : Subsystem
  GEN_R_ADDR_MUX_SEL : Subsystem
  GEN_STB_EOF_W_COUNT : Subsystem
  OUTPUT_MUX : Subsystem
  R_ADDR : Outport
  MUX_SEL : Outport  Port=2
  DOUT : Outport  Port=3
  STB : Outport  Port=4
  EOF : Outport  Port=5
  wires:
  IFG1/1 -> [IFG1]
  IFG0/1 -> [IFG0]
  FEC/1 -> [FEC]
  [EOF] -> EOF/1
  [STB] -> STB/1
  [DOUT] -> DOUT/1
  [MUX_SEL] -> MUX_SEL/1
  [R_ADDR] -> R_ADDR/1
  NODE_ID/1 -> [NODE_ID]
  WE/1 -> [WE]
  DIN/1 -> [DIN]
  NCHAN/1 -> [NCHAN]
  MSYNC/1 -> [MSYNC]
  GEN_R_ADDR_MUX_SEL/2(MUX_SEL) -> [MUX_SEL]
  GEN_R_ADDR_MUX_SEL/1(R_ADDR) -> [R_ADDR]
  OUTPUT_MUX/1(DATA_OUT) -> [DOUT]
  [IFG1] -> OUTPUT_MUX/6(IFG1)
  [IFG0] -> OUTPUT_MUX/5(IFG0)
  [FEC] -> OUTPUT_MUX/4(FEC)
  [NCHAN] -> GEN_R_ADDR_MUX_SEL/3(NCHAN)
  [WE] -> GEN_R_ADDR_MUX_SEL/2(WE)
  [MSYNC] -> GEN_R_ADDR_MUX_SEL/1(MSYNC)
  GEN_STB_EOF_W_COUNT/3(W_COUNT) -> [W_COUNT]
  GEN_STB_EOF_W_COUNT/2(EOF) -> [EOF]
  GEN_STB_EOF_W_COUNT/1(STB) -> [STB]
  [NCHAN] -> GEN_STB_EOF_W_COUNT/3(NCHAN)
  [WE] -> GEN_STB_EOF_W_COUNT/2(WE)
  [MSYNC] -> GEN_STB_EOF_W_COUNT/1(MSYNC)
  [DIN] -> OUTPUT_MUX/3(DATA)
  [ENC_FC] -> OUTPUT_MUX/2(ENC_FC)
  [W_COUNT] -> OUTPUT_MUX/1(W_COUNT)
  GEN_ENC_FC/1(ENC_FC) -> [ENC_FC]
  [EOF] -> GEN_ENC_FC/3(EOF)
  [NODE_ID] -> GEN_ENC_FC/1(NODE_ID)
  [MSYNC] -> GEN_ENC_FC/2(MSYNC)

== system c960x4096_x14_7_r2013b_frb/ds_to_tgbe/mb_wr/MB_WRITE_CNTRS ==
  RESET : Inport
  W_START : Inport  Port=2
  NCHAN : Inport  Port=3
  10_bit_cntr : xbsIndex_r4/Counter  cnt_type=Free Running  cnt_to=Inf  operation=Up  start_count=0  cnt_by_val=1  arith_type=Unsigned  n_bits=10  bin_pt=0  load_pin=off  rst=on  en=on  explicit_period=on  period=1  dbl_ovrd=off  use_behavioral_HDL=off  implementation=Fabric  block_type=counter
  3_bit_cntr : xbsIndex_r4/Counter  cnt_type=Free Running  cnt_to=Inf  operation=Up  start_count=0  cnt_by_val=1  arith_type=Unsigned  n_bits=3  bin_pt=0  load_pin=off  rst=on  en=on  explicit_period=on  period=1  dbl_ovrd=off  use_behavioral_HDL=off  implementation=Fabric  block_type=counter
  4_bit_cntr : xbsIndex_r4/Counter  cnt_type=Free Running  cnt_to=Inf  operation=Up  start_count=0  cnt_by_val=1  arith_type=Unsigned  n_bits=4  bin_pt=0  load_pin=off  rst=on  en=on  explicit_period=on  period=1  dbl_ovrd=off  use_behavioral_HDL=off  implementation=Fabric  block_type=counter
  5_bit_cntr : xbsIndex_r4/Counter  cnt_type=Free Running  cnt_to=Inf  operation=Up  start_count=0  cnt_by_val=1  arith_type=Unsigned  n_bits=5  bin_pt=0  load_pin=off  rst=on  en=on  explicit_period=on  period=1  dbl_ovrd=off  use_behavioral_HDL=off  implementation=Fabric  block_type=counter
  6_bit_cntr : xbsIndex_r4/Counter  cnt_type=Free Running  cnt_to=Inf  operation=Up  start_count=0  cnt_by_val=1  arith_type=Unsigned  n_bits=6  bin_pt=0  load_pin=off  rst=on  en=on  explicit_period=on  period=1  dbl_ovrd=off  use_behavioral_HDL=off  implementation=Fabric  block_type=counter
  7_bit_cntr : xbsIndex_r4/Counter  cnt_type=Free Running  cnt_to=Inf  operation=Up  start_count=0  cnt_by_val=1  arith_type=Unsigned  n_bits=7  bin_pt=0  load_pin=off  rst=on  en=on  explicit_period=on  period=1  dbl_ovrd=off  use_behavioral_HDL=off  implementation=Fabric  block_type=counter
  8_bit_cntr : xbsIndex_r4/Counter  cnt_type=Free Running  cnt_to=Inf  operation=Up  start_count=0  cnt_by_val=1  arith_type=Unsigned  n_bits=8  bin_pt=0  load_pin=off  rst=on  en=on  explicit_period=on  period=1  dbl_ovrd=off  use_behavioral_HDL=off  implementation=Fabric  block_type=counter
  9_bit_cntr : xbsIndex_r4/Counter  cnt_type=Free Running  cnt_to=Inf  operation=Up  start_count=0  cnt_by_val=1  arith_type=Unsigned  n_bits=9  bin_pt=0  load_pin=off  rst=on  en=on  explicit_period=on  period=1  dbl_ovrd=off  use_behavioral_HDL=off  implementation=Fabric  block_type=counter
  Mux : xbsIndex_r4/Mux  inputs=8  en=off  latency=0  precision=Full  arith_type=Unsigned  n_bits=16  bin_pt=14  quantization=Truncate  overflow=Wrap  dbl_ovrd=off  block_type=mux
  ADDR_CNT : Outport
  wires:
  W_START/1 -> 9_bit_cntr/2, 10_bit_cntr/2, 8_bit_cntr/2, 7_bit_cntr/2, 6_bit_cntr/2, 5_bit_cntr/2, 4_bit_cntr/2, 3_bit_cntr/2
  RESET/1 -> 3_bit_cntr/1, 4_bit_cntr/1, 5_bit_cntr/1, 6_bit_cntr/1, 7_bit_cntr/1, 8_bit_cntr/1, 9_bit_cntr/1, 10_bit_cntr/1
  NCHAN/1 -> Mux/1
  Mux/1 -> ADDR_CNT/1
  10_bit_cntr/1 -> Mux/9
  9_bit_cntr/1 -> Mux/8
  8_bit_cntr/1 -> Mux/7
  7_bit_cntr/1 -> Mux/6
  6_bit_cntr/1 -> Mux/5
  5_bit_cntr/1 -> Mux/4
  4_bit_cntr/1 -> Mux/3
  3_bit_cntr/1 -> Mux/2

== system c960x4096_x14_7_r2013b_frb/ds_to_tgbe/mb_wr/MB_WRITE_SLICES ==
  ADDR_CNT : Inport
  NCHAN : Inport  Port=2
  ADDR_1 : Subsystem
  ADDR_128 : Subsystem
  ADDR_16 : Subsystem
  ADDR_2 : Subsystem
  ADDR_32 : Subsystem
  ADDR_4 : Subsystem
  ADDR_64 : Subsystem
  ADDR_8 : Subsystem
  Mux : xbsIndex_r4/Mux  inputs=8  en=off  latency=0  precision=Full  arith_type=Unsigned  n_bits=16  bin_pt=14  quantization=Truncate  overflow=Wrap  dbl_ovrd=off  block_type=mux
  W_ADDR : Outport
  wires:
  Mux/1 -> W_ADDR/1
  ADDR_CNT/1 -> ADDR_1/1(ADDR_CNT), ADDR_2/1(ADDR_CNT), ADDR_4/1(ADDR_CNT), ADDR_8/1(ADDR_CNT), ADDR_16/1(ADDR_CNT), ADDR_32/1(ADDR_CNT), ADDR_64/1(ADDR_CNT), ADDR_128/1(ADDR_CNT)
  NCHAN/1 -> Mux/1
  ADDR_128/1(W_ADDR) -> Mux/9
  ADDR_64/1(W_ADDR) -> Mux/8
  ADDR_32/1(W_ADDR) -> Mux/7
  ADDR_16/1(W_ADDR) -> Mux/6
  ADDR_8/1(W_ADDR) -> Mux/5
  ADDR_4/1(W_ADDR) -> Mux/4
  ADDR_2/1(W_ADDR) -> Mux/3
  ADDR_1/1(W_ADDR) -> Mux/2

== system c960x4096_x14_7_r2013b_frb/ds_to_tgbe/mb_wr/START_LATCH ==
  RESET : Inport
  SET : Inport  Port=2
  Logical : xbsIndex_r4/Logical  logical_function=OR  inputs=2  en=off  latency=0  precision=Full  arith_type=Unsigned  n_bits=16  bin_pt=0  align_bp=on  dbl_ovrd=off  block_type=logical
  Register : xbsIndex_r4/Register  init=0  rst=on  en=off  dbl_ovrd=off  block_type=register
  OUT : Outport
  wires:
  SET/1 -> Logical/2
  RESET/1 -> Register/2
  Register/1 -> OUT/1, Logical/1
  Logical/1 -> Register/1

== system c960x4096_x14_7_r2013b_frb/ds_to_tgbe/mb_wr/WE_DECODE_BITS ==
  ADDR_CNT : Inport
  NCHAN : Inport  Port=2
  Mux : xbsIndex_r4/Mux  inputs=8  en=off  latency=0  precision=Full  arith_type=Unsigned  n_bits=16  bin_pt=14  quantization=Truncate  overflow=Wrap  dbl_ovrd=off  block_type=mux
  Slice_bits_210 : xbsIndex_r4/Slice  nbits=3  boolean_output=off  mode=Upper Bit Location + Width  bit1=-7  base1=MSB of Input  bit0=0  base0=LSB of Input  dbl_ovrd=off  block_type=slice
  Slice_bits_321 : xbsIndex_r4/Slice  nbits=3  boolean_output=off  mode=Upper Bit Location + Width  bit1=-6  base1=MSB of Input  bit0=0  base0=LSB of Input  dbl_ovrd=off  block_type=slice
  Slice_bits_432 : xbsIndex_r4/Slice  nbits=3  boolean_output=off  mode=Upper Bit Location + Width  bit1=-5  base1=MSB of Input  bit0=0  base0=LSB of Input  dbl_ovrd=off  block_type=slice
  Slice_bits_543 : xbsIndex_r4/Slice  nbits=3  boolean_output=off  mode=Upper Bit Location + Width  bit1=-4  base1=MSB of Input  bit0=0  base0=LSB of Input  dbl_ovrd=off  block_type=slice
  Slice_bits_654 : xbsIndex_r4/Slice  nbits=3  boolean_output=off  mode=Upper Bit Location + Width  bit1=-3  base1=MSB of Input  bit0=0  base0=LSB of Input  dbl_ovrd=off  block_type=slice
  Slice_bits_765 : xbsIndex_r4/Slice  nbits=3  boolean_output=off  mode=Upper Bit Location + Width  bit1=-2  base1=MSB of Input  bit0=0  base0=LSB of Input  dbl_ovrd=off  block_type=slice
  Slice_bits_876 : xbsIndex_r4/Slice  nbits=3  boolean_output=off  mode=Upper Bit Location + Width  bit1=-1  base1=MSB of Input  bit0=0  base0=LSB of Input  dbl_ovrd=off  block_type=slice
  Slice_bits_987 : xbsIndex_r4/Slice  nbits=3  boolean_output=off  mode=Upper Bit Location + Width  bit1=0  base1=MSB of Input  bit0=0  base0=LSB of Input  dbl_ovrd=off  block_type=slice
  WE_DECODE : Outport
  wires:
  Mux/1 -> WE_DECODE/1
  ADDR_CNT/1 -> Slice_bits_210/1, Slice_bits_321/1, Slice_bits_432/1, Slice_bits_543/1, Slice_bits_654/1, Slice_bits_765/1, Slice_bits_876/1, Slice_bits_987/1
  NCHAN/1 -> Mux/1
  Slice_bits_210/1 -> Mux/2
  Slice_bits_321/1 -> Mux/3
  Slice_bits_432/1 -> Mux/4
  Slice_bits_543/1 -> Mux/5
  Slice_bits_654/1 -> Mux/6
  Slice_bits_765/1 -> Mux/7
  Slice_bits_876/1 -> Mux/8
  Slice_bits_987/1 -> Mux/9

== system c960x4096_x14_7_r2013b_frb/leds/Pulse_Ext/edge_detect ==
  in : Inport
  Delay : xbsIndex_r4/Delay  rst=off  infoeditControl=Selection of Reset will increase slice count due to use of real FFs and instead of SRLs  en=off  latency=1  dbl_ovrd=off  reg_retiming=off  block_type=delay
      settings: xl_area=[0, 0, 0, 0, 0, 0, 0]
  Inverter : xbsIndex_r4/Inverter  en=off  latency=0  dbl_ovrd=off  block_type=inv
      settings: xl_area=[0, 0, 0, 0, 0, 0, 0]
  edge_op : xbsIndex_r4/Logical  logical_function=NOR  inputs=2  en=off  latency=0  precision=Full  arith_type=Unsigned  n_bits=8  bin_pt=2  align_bp=on  dbl_ovrd=off  block_type=logical
      settings: xl_area=[0, 0, 0, 0, 0, 0, 0]
  out : Outport
  wires:
  Inverter/1 -> edge_op/1
  edge_op/1 -> out/1
  in/1 -> Inverter/1, Delay/1
  Delay/1 -> edge_op/2

== system c960x4096_x14_7_r2013b_frb/leds/Pulse_Ext1/edge_detect ==
  in : Inport
  Delay : xbsIndex_r4/Delay  rst=off  infoeditControl=Selection of Reset will increase slice count due to use of real FFs and instead of SRLs  en=off  latency=1  dbl_ovrd=off  reg_retiming=off  block_type=delay
      settings: xl_area=[0, 0, 0, 0, 0, 0, 0]
  Inverter : xbsIndex_r4/Inverter  en=off  latency=0  dbl_ovrd=off  block_type=inv
      settings: xl_area=[0, 0, 0, 0, 0, 0, 0]
  edge_op : xbsIndex_r4/Logical  logical_function=NOR  inputs=2  en=off  latency=0  precision=Full  arith_type=Unsigned  n_bits=8  bin_pt=2  align_bp=on  dbl_ovrd=off  block_type=logical
      settings: xl_area=[0, 0, 0, 0, 0, 0, 0]
  out : Outport
  wires:
  Inverter/1 -> edge_op/1
  edge_op/1 -> out/1
  in/1 -> Inverter/1, Delay/1
  Delay/1 -> edge_op/2
